simulink model "lmt86"  (R2021a)
settings: Solver=VariableStepAuto  StartTime=0.0  StopTime=10.0  RelTol=1e-3
settings Model: Creator=Yusuf  LastModifiedBy=Yusuf

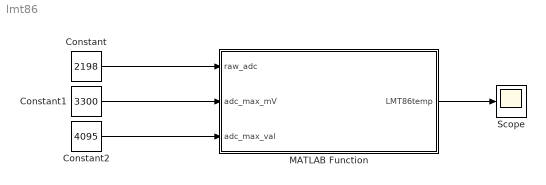
== system lmt86 ==
  Constant : Constant  Value=2198
  Constant1 : Constant  Value=3300
  Constant2 : Constant  Value=4095
  MATLAB Function : MATLAB Function  TreatAsAtomicUnit=on
  Scope : Scope
  wires:
  Constant2/1 -> MATLAB Function/3(adc_max_val)
  Constant1/1 -> MATLAB Function/2(adc_max_mV)
  Constant/1 -> MATLAB Function/1(raw_adc)
  MATLAB Function/1(LMT86temp) -> Scope/1

== matlab function lmt86/MATLAB Function ==
  data: raw_adc input; LMT86temp output; adc_max_mV input; adc_max_val input
function LMT86temp = ADCtoCelcius(raw_adc, adc_max_mV, adc_max_val)

voltage = (adc_max_mV / adc_max_val) * raw_adc;
temp = ((10.888 - sqrt( (-10.888)^2 + 4 * 0.00347 * (1777.3 - voltage) )) / (2 * (-0.00347))) + 30;

LMT86temp = temp;
